simulink model "vcu_0110"  (R2024b)
settings: Solver=FixedStepAuto  StartTime=0.0  StopTime=2000  FixedStep=0.001  RelTol=1e-3
libraries: canoelib x13, sim3dautolib x2, sim3dlib x1
settings Model: Creator=USER  LastModifiedBy=USER
settings DebuggingCC: AlgebraicLoopMsg=none

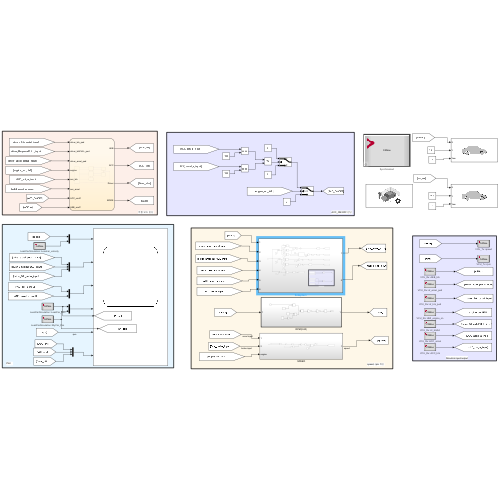
[thumbnail: Simulink's stored preview of the top-level diagram]
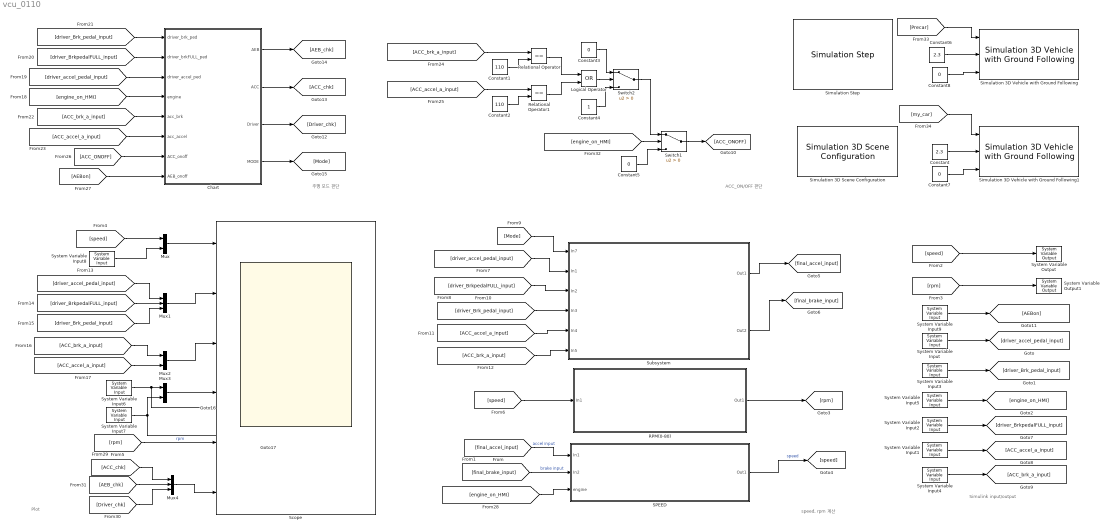
== system vcu_0110 ==
  note: Simulink input/output
  note: ACC_ON/OFF 판단
  note: Plot
  note: 주행 모드 판단
  note: speed, rpm 계산
  Chart : Stateflow chart  TreatAsAtomicUnit=on
      settings: PortSchema="{\"entries\":[{\"content\":{\"sides\":[{\"content\":{},\"type\":\"ConnectorPlacement.EquallySpacedRectSide\",\"uuid\":\"820ebdc8-5d3c-4f1f-b280-fea0b50c545f\"},{\"content\":{\"side\":\"RIGHT\"},\"type\":\"ConnectorPlacement.EquallySpacedRectSide\",\"uuid\":\"46a8381c-917c-43fc-9903-c651e2f7d6ed\"},{\"content\":{\"connectorIds\":[\"In1\",\"In2\",\"In3\",\"In4\",\"In5\",\"In6\",\"In7\",\"In8\"],\"side\":\"TOP\"},\"type\":\"ConnectorPlacement.EquallySpacedRectSide\",\"uuid\":\"b91c132f-a4fd-45a1-86f9-b94de235e8d0\"},{\"content\":{\"connectorIds\":[\"Out1\",\"Out2\",\"Out3\",\"Out4\"],\"side\":\"BOTTOM\"},\"type\":\"ConnectorPlacement.EquallySpacedRectSide\",\"uuid\":\"00e0a422-08e9-4016-b93b-daa058c76a47\"}]},\"type\":\"ConnectorPlacement.EquallySpacedConnector\",\"uuid\":\"f2db09bc-dfcd-4890-8deb-cb96adcd2283\"}],\"packageUris\":[\"http://schema.mathworks.com/mf0/Connector/R2020b\"],\"version\":\"1.0\"}"
  Constant : Constant  Value=2.3
  Constant1 : Constant  Value=110
  Constant2 : Constant  Value=110
  Constant{3,5,7..8} (4 alike) : Constant  Value=0
  Constant4 : Constant
  Constant6 : Constant  Value=2.3
  Logical Operator : Logic  Operator=OR  AllPortsSameDT=off  OutDataTypeStr=boolean
  Mux : Mux  Inputs=2
  Mux1 : Mux  Inputs=3
  Mux2 : Mux  Inputs=2
  Mux3 : Mux  Inputs=2
  Mux4 : Mux  Inputs=3
  RPM(0-80) : Subsystem  TreatAsAtomicUnit=on  SystemSampleTime=1
  Relational Operator : RelationalOperator  Operator===  OutDataTypeStr=boolean  RndMeth=Simplest  InputSameDT=off
  Relational Operator1 : RelationalOperator  Operator===  OutDataTypeStr=boolean  RndMeth=Simplest  InputSameDT=off
  SPEED : Subsystem
  Scope : Scope  NumInputPorts=6
  Simulation 3D Scene Configuration : sim3dlib/Simulation 3D Scene Configuration  Priority=0  ProjectFormat=Default Scenes  SceneDesc=Straight road  ProjectName=C:\Program Files\MATLAB\R2024b\toolbox\shared\sim3d_projects\automotive_project_windows\UE\WindowsNoEditor\VehicleSimulation.exe  ScenePath=/Game/Maps/HwStrght  EnableOpenDRIVE=off  vehTagList={'Custom';'Scene Origin';'SimulinkVehicle1';'SimulinkVehicle2'}  vehTag=SimulinkVehicle1  FreeCameraInitialTranslation=[50, 0, 200]  FreeCameraDefaultInitialTranslation=[-6, 0, 2]  FreeCameraInitialRotation=[0, -90, 0]  FreeCameraDefaultInitialRotation=[0, -15, 0]  OpVisEn=off  Ts=.02  EnableWindow=on  EnableRemoteAccess=off  EnableWeather=off  SunAzimuth=90  SunAltitude=40.0  EnableGeospatialSun=off  Latitude=0  Longitude=0  Date=2023-01-01  Time=10:30:00  GeoTimeZone=-5.0  SunDaylightSaving=off  wind=1  clouds=10  EnableVolumetricClouds=off  CloudCoverage=0  CloudAltitude=6  fog=0  rain=0  RaindropsEffect=off  SnowDensity=0  EnableGeospatial=off  UseTrueOrigin=off  OriginHeight=200  OriginLatitude=40.744652  OriginLongitude=-73.988864  MapStyle=Aerial  AdditionalAssetIDs=[]  UseAdvancedSunSky=off  SolarTime=11  TimeZone=-5  Day=21  Month=9  Year=2022  UseDaylightSavingTime=on  DSTStartDay=10  DSTStartMonth=3  DSTEndDay=3  DSTEndMonth=11  DSTSwitchHour=2  sensorTag=MainCamera1  sensorId=1  sensorName=MainCamera1  mountLoc=Origin  offsetFlag=off  tmountOffset=[0, 0, 0]  rmountOffset=[0, 0, 0]  HorizontalResolution=1280  VerticalResolution=720  HorizontalFOV=60  mountPoint=[0 0 0]  mountOrientation=[0 0 0]  aMode=5  ID=1  GeoTrigger=Inactive
      settings: LibrarySourceBlock=sl3dlib/Simulation 3D/Environment/Simulation 3D Scene Configuration
  Simulation 3D Vehicle with Ground Following : sim3dautolib/Simulation 3D Vehicle with Ground Following  Priority=1  PassVehMesh=Muscle car  MeshPath=/MathWorksAutomotiveContent/Vehicles/Muscle/Meshes/SK_MuscleCar.SK_MuscleCar  TrackWidth=1.9  WheelBase=3  WheelRadius=0.35  VehColor=Green  InitialPos=[0, 0, 0]  InitialRot=[0, 0, 0]  ActorName=SimulinkVehicle2  SampleTime=-1  ActorType=SimulinkVehicle  ID=2  aMode=5  ActorTag=SimulinkVehicle2  CoordinateScheme=ISO  VehLightsControl=off  HeadlightColor=[ 1, 1, 1 ]  HighBeamIntensity=100000  LowBeamIntensity=60000  HighBeamConeAngle=70  LowBeamConeAngle=70  LeftHeadlightOrientation=[ 0, 0 ]  RightHeadlightOrientation=[ 0, 0 ]  BrakelightIntensity=500  ReverselightIntensity=500  SignallightIntensity=500  SignallightPeriod=1  SignalPulseWidth=50  TransformOutportEnabled=off
      settings: LibrarySourceBlock=sl3dlib/Simulation 3D/Actors/Simulation 3D Vehicle with Ground Following
  Simulation 3D Vehicle with Ground Following1 : sim3dautolib/Simulation 3D Vehicle with Ground Following  Priority=1  PassVehMesh=Muscle car  MeshPath=/MathWorksAutomotiveContent/Vehicles/Muscle/Meshes/SK_MuscleCar.SK_MuscleCar  TrackWidth=1.9  WheelBase=3  WheelRadius=0.35  VehColor=Red  InitialPos=[0, 0, 0]  InitialRot=[0, 0, 0]  ActorName=SimulinkVehicle1  SampleTime=-1  ActorType=SimulinkVehicle  ID=1  aMode=5  ActorTag=SimulinkVehicle1  CoordinateScheme=ISO  VehLightsControl=off  HeadlightColor=[ 1, 1, 1 ]  HighBeamIntensity=100000  LowBeamIntensity=60000  HighBeamConeAngle=70  LowBeamConeAngle=70  LeftHeadlightOrientation=[ 0, 0 ]  RightHeadlightOrientation=[ 0, 0 ]  BrakelightIntensity=500  ReverselightIntensity=500  SignallightIntensity=500  SignallightPeriod=1  SignalPulseWidth=50  TransformOutportEnabled=off
      settings: LibrarySourceBlock=sl3dlib/Simulation 3D/Actors/Simulation 3D Vehicle with Ground Following
  Simulation Step : canoelib/CANoe I//O/Simulation Step  mode=Synchronized
      settings: AttributesFormatString=%<mode>  SourceProductName=Vector CANoe
  Subsystem : Subsystem
  Switch1 : Switch  Criteria=u2 > Threshold  SaturateOnIntegerOverflow=off  InputSameDT=off
  Switch2 : Switch  Criteria=u2 > Threshold  SaturateOnIntegerOverflow=off  InputSameDT=off
  System Variable Input : canoelib/CANoe I//O/System Variable Input  nsName=VCU_Rx  sysVarName=dr_accel_ped  arrayIndex=-1  editSampleTime=0  rawValue=Default  dataType=Default  dataTypeDB=int32  hasEncoding=off  dataTypeCANoe=Get from CANoe
      settings: AttributesFormatString=%<nsName>::%<sysVarName>  SourceProductName=Vector CANoe
  System Variable Input1 : canoelib/CANoe I//O/System Variable Input  nsName=VCU_Rx  sysVarName=ACC_accel  arrayIndex=-1  editSampleTime=0  rawValue=Default  dataType=Default  dataTypeDB=int32  hasEncoding=off  dataTypeCANoe=Get from CANoe
      settings: AttributesFormatString=%<nsName>::%<sysVarName>  SourceProductName=Vector CANoe
  System Variable Input2 : canoelib/CANoe I//O/System Variable Input  nsName=VCU_Rx  sysVarName=dr_brkfull  arrayIndex=-1  editSampleTime=0  rawValue=Default  dataType=Default  dataTypeDB=int32  hasEncoding=off  dataTypeCANoe=Get from CANoe
      settings: AttributesFormatString=%<nsName>::%<sysVarName>  SourceProductName=Vector CANoe
  System Variable Input3 : canoelib/CANoe I//O/System Variable Input  nsName=VCU_Rx  sysVarName=dr_brk_ped  arrayIndex=-1  editSampleTime=0  rawValue=Default  dataType=Default  dataTypeDB=int32  hasEncoding=off  dataTypeCANoe=Get from CANoe
      settings: AttributesFormatString=%<nsName>::%<sysVarName>  SourceProductName=Vector CANoe
  System Variable Input4 : canoelib/CANoe I//O/System Variable Input  nsName=VCU_Rx  sysVarName=ACC_brk  arrayIndex=-1  editSampleTime=0  rawValue=Default  dataType=Default  dataTypeDB=int32  hasEncoding=off  dataTypeCANoe=Get from CANoe
      settings: AttributesFormatString=%<nsName>::%<sysVarName>  SourceProductName=Vector CANoe
  System Variable Input5 : canoelib/CANoe I//O/System Variable Input  nsName=VCU_Rx  sysVarName=HMI_engine_on  arrayIndex=-1  editSampleTime=0  rawValue=Default  dataType=Default  dataTypeDB=int32  hasEncoding=off  dataTypeCANoe=Get from CANoe
      settings: AttributesFormatString=%<nsName>::%<sysVarName>  SourceProductName=Vector CANoe
  System Variable Input6 : canoelib/CANoe I//O/System Variable Input  nsName=LeadCarSimulation  sysVarName=LeadCar_Pos  arrayIndex=-1  editSampleTime=0  rawValue=Default  dataType=Default  dataTypeDB=double  hasEncoding=off  dataTypeCANoe=Get from CANoe
      settings: AttributesFormatString=%<nsName>::%<sysVarName>  SourceProductName=Vector CANoe
  System Variable Input7 : canoelib/CANoe I//O/System Variable Input  nsName=LeadCarSimulation  sysVarName=MyCar_Pos  arrayIndex=-1  editSampleTime=0  rawValue=Default  dataType=Default  dataTypeDB=double  hasEncoding=off  dataTypeCANoe=Get from CANoe
      settings: AttributesFormatString=%<nsName>::%<sysVarName>  SourceProductName=Vector CANoe
  System Variable Input8 : canoelib/CANoe I//O/System Variable Input  nsName=LeadCarSimulation  sysVarName=Leadcar_velocity  arrayIndex=-1  editSampleTime=0  rawValue=Default  dataType=Default  dataTypeDB=int32  hasEncoding=off  dataTypeCANoe=Get from CANoe
      settings: AttributesFormatString=%<nsName>::%<sysVarName>  SourceProductName=Vector CANoe
  System Variable Input9 : canoelib/CANoe I//O/System Variable Input  nsName=VCU_Rx  sysVarName=AEB_brk  arrayIndex=-1  editSampleTime=0  rawValue=Default  dataType=Default  dataTypeDB=int32  hasEncoding=off  dataTypeCANoe=Get from CANoe
      settings: AttributesFormatString=%<nsName>::%<sysVarName>  SourceProductName=Vector CANoe
  System Variable Output : canoelib/CANoe I//O/System Variable Output  nsName=VCU_Tx  sysVarName=speed  arrayIndex=-1  rawValue=Default  dataType=Default  dataTypeDB=int32  hasEncoding=off  dataTypeCANoe=Get from CANoe
      settings: AttributesFormatString=%<nsName>::%<sysVarName>  SourceProductName=Vector CANoe
  System Variable Output1 : canoelib/CANoe I//O/System Variable Output  nsName=VCU_Tx  sysVarName=rpm  arrayIndex=-1  rawValue=Default  dataType=Default  dataTypeDB=int32  hasEncoding=off  dataTypeCANoe=Get from CANoe
      settings: AttributesFormatString=%<nsName>::%<sysVarName>  SourceProductName=Vector CANoe
  wires:
  [rpm] -> System Variable Output1/1
  [final_accel_input] -> SPEED/1(In1)  "accel input"
  [final_brake_input] -> SPEED/2(In2)  "brake input"
  SPEED/1(Out1) -> [speed]  "speed"
  [speed] -> RPM(0-80)/1(In1)
  RPM(0-80)/1(Out1) -> [rpm]
  [driver_accel_pedal_input] -> Subsystem/2(In1)
  [driver_Brk_pedal_input] -> Subsystem/4(In3)
  Subsystem/2(Out2) -> [final_brake_input]
  Subsystem/1(Out1) -> [final_accel_input]
  System Variable Input/1 -> [driver_accel_pedal_input]
  System Variable Input3/1 -> [driver_Brk_pedal_input]
  System Variable Input5/1 -> [engine_on_HMI]
  [driver_BrkpedalFULL_input] -> Subsystem/3(In2)
  System Variable Input2/1 -> [driver_BrkpedalFULL_input]
  System Variable Input1/1 -> [ACC_accel_a_input]
  System Variable Input4/1 -> [ACC_brk_a_input]
  [ACC_brk_a_input] -> Subsystem/6(In5)
  [speed] -> System Variable Output/1
  [driver_accel_pedal_input] -> Mux1/1
  [driver_BrkpedalFULL_input] -> Mux1/2
  [driver_Brk_pedal_input] -> Mux1/3
  [ACC_brk_a_input] -> Mux2/1
  [ACC_accel_a_input] -> Mux2/2
  [speed] -> Mux/1
  [rpm] -> Scope/5  "rpm"
  Mux/1 -> Scope/1
  Mux1/1 -> Scope/2
  Mux2/1 -> Scope/3
  [ACC_accel_a_input] -> Subsystem/5(In4)
  System Variable Input6/1 -> [Precar], Mux3/1
  Mux3/1 -> Scope/4
  System Variable Input7/1 -> [my_car], Mux3/2
  System Variable Input8/1 -> Mux/2
  [engine_on_HMI] -> Chart/5(engine)
  [ACC_brk_a_input] -> Chart/4(acc_brk)
  [ACC_accel_a_input] -> Chart/3(acc_accel)
  Constant1/1 -> Relational Operator/2
  [ACC_accel_a_input] -> Relational Operator1/1
  Constant2/1 -> Relational Operator1/2
  Relational Operator/1 -> Logical Operator/1
  Relational Operator1/1 -> Logical Operator/2
  Logical Operator/1 -> Switch2/2
  Constant3/1 -> Switch2/1
  Constant4/1 -> Switch2/3
  [ACC_ONOFF] -> Chart/2(ACC_onoff)
  System Variable Input9/1 -> [AEBon]
  [AEBon] -> Chart/1(AEB_onoff)
  Chart/3(ACC) -> [ACC_chk]
  Chart/2(Driver) -> [Driver_chk]
  Chart/4(AEB) -> [AEB_chk]
  Chart/1(MODE) -> [Mode]
  [Mode] -> Subsystem/1(In7)
  [engine_on_HMI] -> SPEED/3(engine)
  Mux4/1 -> Scope/6
  [ACC_chk] -> Mux4/1
  [AEB_chk] -> Mux4/2
  [Driver_chk] -> Mux4/3
  [driver_accel_pedal_input] -> Chart/6(driver_accel_ped)
  [driver_BrkpedalFULL_input] -> Chart/7(driver_brkFULL_ped)
  [driver_Brk_pedal_input] -> Chart/8(driver_brk_ped)
  [ACC_brk_a_input] -> Relational Operator/1
  [engine_on_HMI] -> Switch1/2
  Constant5/1 -> Switch1/3
  Switch2/1 -> Switch1/1
  Switch1/1 -> [ACC_ONOFF]
  Constant/1 -> Simulation 3D Vehicle with Ground Following1/2
  Constant6/1 -> Simulation 3D Vehicle with Ground Following/2
  [my_car] -> Simulation 3D Vehicle with Ground Following1/1
  [Precar] -> Simulation 3D Vehicle with Ground Following/1
  Constant7/1 -> Simulation 3D Vehicle with Ground Following1/3
  Constant8/1 -> Simulation 3D Vehicle with Ground Following/3

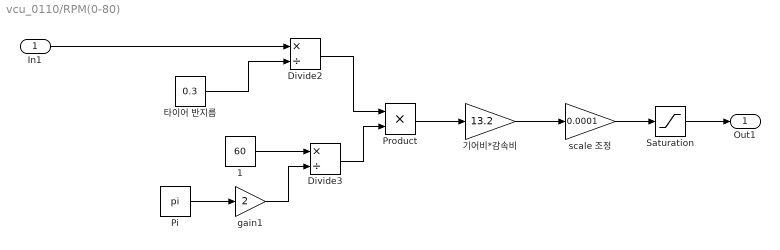
== system vcu_0110/RPM(0-80) ==
  In1 : Inport
  " 1" : Constant  Value=60
  Divide2 : Product  Inputs=*/
  Divide3 : Product  Inputs=*/
  Pi : Constant  Value=pi  OutDataTypeStr=Inherit: Inherit via back propagation
  Product : Product
  Saturation : Saturate  UpperLimit=8  LowerLimit=1
  gain1 : Gain  Gain=2
  scale 조정 : Gain  Gain=0.0001
  기어비*감속비 : Gain  Gain=13.2
  타이어 반지름 : Constant  Value=0.3
  Out1 : Outport
  wires:
  기어비*감속비/1 -> scale 조정/1
  " 1"/1 -> Divide3/1
  Pi/1 -> gain1/1
  Divide3/1 -> Product/2
  Divide2/1 -> Product/1
  gain1/1 -> Divide3/2
  타이어 반지름/1 -> Divide2/2
  Product/1 -> 기어비*감속비/1
  In1/1 -> Divide2/1
  scale 조정/1 -> Saturation/1
  Saturation/1 -> Out1/1

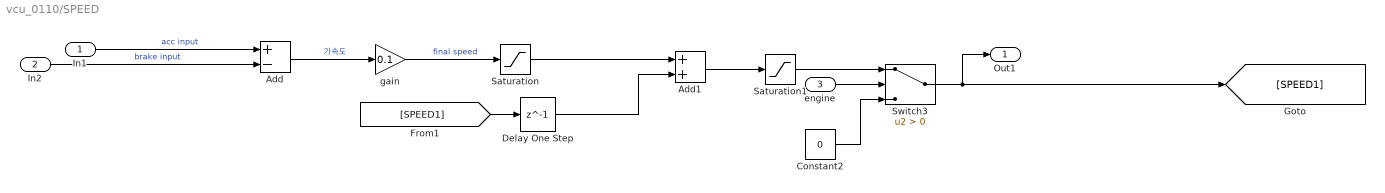
== system vcu_0110/SPEED ==
  In1 : Inport
  In2 : Inport  Port=2
  engine : Inport  Port=3
  Add : Sum  Inputs=+-
  Add1 : Sum
  Constant2 : Constant  Value=0
  Delay One Step : Delay  DelayLength=1
  Saturation : Saturate  UpperLimit=10  LowerLimit=-5
  Saturation1 : Saturate  UpperLimit=250  LowerLimit=0
  Switch3 : Switch  Criteria=u2 > Threshold  SaturateOnIntegerOverflow=off  InputSameDT=off
  gain : Gain  Gain=0.1
  Out1 : Outport
  wires:
  Add/1 -> gain/1  "가속도"
  Saturation/1 -> Add1/1
  gain/1 -> Saturation/1  "final speed"
  In1/1 -> Add/1  "acc input"
  [SPEED1] -> Delay One Step/1
  Delay One Step/1 -> Add1/2
  Add1/1 -> Saturation1/1
  engine/1 -> Switch3/2
  Saturation1/1 -> Switch3/1
  Constant2/1 -> Switch3/3
  Switch3/1 -> Out1/1, [SPEED1]
  In2/1 -> Add/2  "brake input"

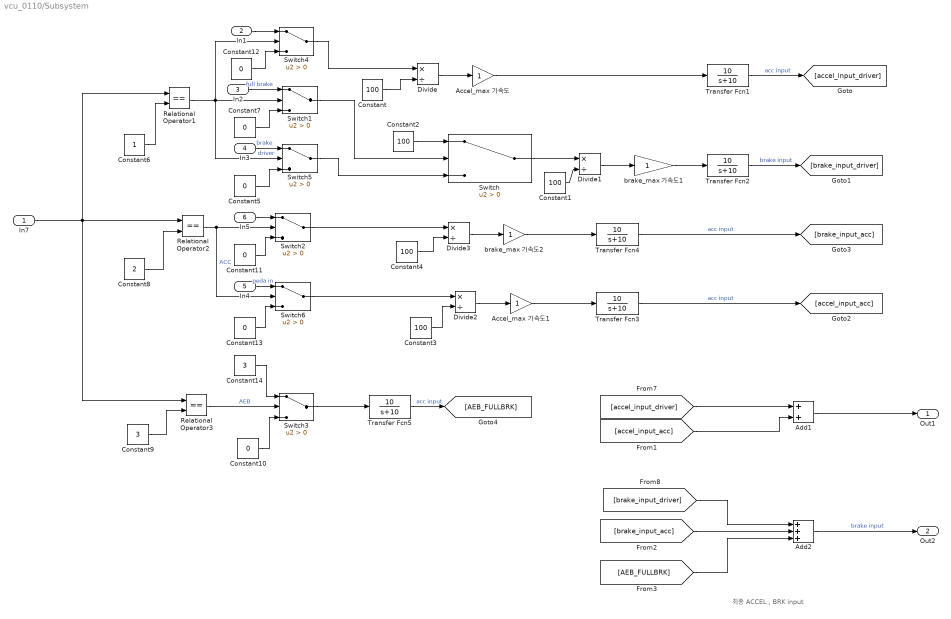
== system vcu_0110/Subsystem ==
  note: 최종 ACCEL , BRK input
  In7 : Inport
  In1 : Inport  Port=2
  In2 : Inport  Port=3
  In3 : Inport  Port=4
  In4 : Inport  Port=5
  In5 : Inport  Port=6
  Accel_max 가속도 : Gain
  Accel_max 가속도1 : Gain
  Add1 : Sum
  Add2 : Sum  Inputs=+++
  Constant{,1..4} (5 alike) : Constant  Value=100
  Constant{5,7,10..13} (6 alike) : Constant  Value=0
  Constant14 : Constant  Value=3
  Constant6 : Constant
  Constant8 : Constant  Value=2
  Constant9 : Constant  Value=3
  Divide{,1..3} (4 alike) : Product  Inputs=*/
  Relational Operator1 : RelationalOperator  Operator===  OutDataTypeStr=boolean  RndMeth=Simplest  InputSameDT=off
  Relational Operator2 : RelationalOperator  Operator===  OutDataTypeStr=boolean  RndMeth=Simplest  InputSameDT=off
  Relational Operator3 : RelationalOperator  Operator===  OutDataTypeStr=boolean  RndMeth=Simplest  InputSameDT=off
  Switch{,1..6} (7 alike) : Switch  Criteria=u2 > Threshold  SaturateOnIntegerOverflow=off  InputSameDT=off
  Transfer Fcn{1..5} (5 alike) : TransferFcn  Numerator=[10]  Denominator=[1 10]
  brake_max 가속도1 : Gain
  brake_max 가속도2 : Gain
  Out1 : Outport
  Out2 : Outport  Port=2
  wires:
  Constant/1 -> Divide/2
  Constant1/1 -> Divide1/2
  [accel_input_driver] -> Add1/1
  [brake_input_driver] -> Add2/1
  brake_max 가속도1/1 -> Transfer Fcn2/1
  Divide/1 -> Accel_max 가속도/1
  Divide1/1 -> brake_max 가속도1/1
  Switch/1 -> Divide1/1
  Constant2/1 -> Switch/1
  Add1/1 -> Out1/1
  Transfer Fcn1/1 -> [accel_input_driver]  "acc input"
  Transfer Fcn2/1 -> [brake_input_driver]  "brake input"
  Accel_max 가속도/1 -> Transfer Fcn1/1
  Accel_max 가속도1/1 -> Transfer Fcn3/1
  Transfer Fcn3/1 -> [accel_input_acc]  "acc input"
  Constant3/1 -> Divide2/2
  Divide2/1 -> Accel_max 가속도1/1
  [accel_input_acc] -> Add1/2
  Divide3/1 -> brake_max 가속도2/1
  Constant4/1 -> Divide3/2
  brake_max 가속도2/1 -> Transfer Fcn4/1
  Transfer Fcn4/1 -> [brake_input_acc]  "acc input"
  [brake_input_acc] -> Add2/2
  In7/1 -> Relational Operator3/1, Relational Operator1/1, Relational Operator2/1
  Constant6/1 -> Relational Operator1/2
  Constant7/1 -> Switch1/3
  Constant8/1 -> Relational Operator2/2
  Constant9/1 -> Relational Operator3/2
  Relational Operator2/1 -> Switch6/2, Switch2/2  "ACC"
  Relational Operator3/1 -> Switch3/2  "AEB"
  Constant10/1 -> Switch3/3
  Constant11/1 -> Switch2/3
  Constant12/1 -> Switch4/3
  In1/1 -> Switch4/1
  Switch4/1 -> Divide/1
  Constant5/1 -> Switch5/3
  Relational Operator1/1 -> Switch5/2, Switch4/2, Switch1/2  "driver"
  In2/1 -> Switch1/1  "full brake"
  Switch1/1 -> Switch/2
  In3/1 -> Switch5/1  "brake"
  Switch5/1 -> Switch/3
  In5/1 -> Switch2/1
  Switch2/1 -> Divide3/1
  Constant13/1 -> Switch6/3
  In4/1 -> Switch6/1  "peda in"
  Switch6/1 -> Divide2/1
  Constant14/1 -> Switch3/1
  Switch3/1 -> Transfer Fcn5/1
  Transfer Fcn5/1 -> [AEB_FULLBRK]  "acc input"
  [AEB_FULLBRK] -> Add2/3
  Add2/1 -> Out2/1  "brake input"

== stateflow chart vcu_0110/Chart ==
  state Init
    en:
    ACC=0;
    Driver=0;
    AEB=0;
    MODE=0;
  state Driver_M
    en:
    ACC=0;
    Driver=1;
    AEB=0;
    MODE=1;
    DRcnt = uint16(1);
    du:
    DRcnt =DRcnt+1;
    ex:DRcnt=uint16(0)
  state AEB_wDriver
    en:
    ACC=0;
    Driver=0;
    AEB=1;
    MODE=3;
  note: 값이 튀는경우 방지
  state ACC_M
    en:
    ACC=1;
    Driver=0;
    AEB=0;
    MODE=2;
    ACCnt = uint16(1);
    du:
    ACCnt =ACCnt+1;
    ex:ACCnt=uint16(0)
  note: (ACCnt <3 && acc_accel ==0 || ACCnt <3 && acc_brk==0)
  state AEB_wACC
    en:
    ACC=0;
    Driver=0;
    AEB=1;
    MODE=3;
  state Driver_wACC
    en:
    ACC=0;
    Driver=1;
    AEB=0;
    MODE=1;
  (default) -> Init
  Init -> Driver_M [order 1] : [ (engine==1 && ACC_onoff == 0)
      | ]
  Driver_M -> AEB_wDriver [order 2] : [AEB_onoff ==1]
  Driver_M -> Init [order 3] : [engine==0]
  AEB_wDriver -> Driver_M [order 1] : [AEB_onoff ==0]
  ACC_M -> Driver_M [order 4] : [ (engine ==1 && ACC_onoff ==0) ||...
      | (driver_brk_ped >0 || driver_brkFULL_ped > 0 ) ]
  Driver_M -> ACC_M [order 1] : [ACC_onoff ==1&& DRcnt >=2]
  AEB_wDriver -> (junction 42) [order 2] : [engine==0]
  (junction 42) -> (junction 45)
  AEB_wACC -> (junction 42) [order 2] : [engine==0]
  (junction 45) -> (junction 47)
  Init -> ACC_M [order 2] : [ (engine==1 &&   ACC_onoff ==1) ]
  AEB_wACC -> ACC_M [order 1] : [AEB_onoff ==0]
  ACC_M -> Init [order 1] : [engine==0 && ACC_onoff ==0]
  ACC_M -> AEB_wACC [order 2] : [AEB_onoff ==1]
  ACC_M -> Driver_wACC [order 3] : [driver_accel_ped >0]
  Driver_wACC -> ACC_M [order 1] : [driver_accel_ped == 0]
  Driver_wACC -> Init [order 2] : [engine==0 ]
  (junction 47) -> Init
  data: MODE output; Driver output; AEB_onoff input; ACC_onoff input; acc_accel input; acc_brk input; ACC output; AEB output; engine input; driver_accel_ped input; driver_brkFULL_ped input; driver_brk_ped input; ACCnt local; DRcnt local
